simulink model "BillardSchieftischOneBall"  (Simulink 7.1)
settings: Solver=ode45  StartTime=0.0  StopTime=15.0  RelTol=1e-3
libraries: simulink x1
settings Model: Creator=Meisel  LastModifiedBy=Meisel

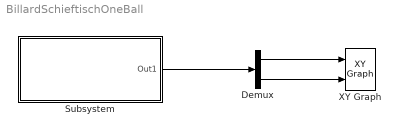
== system BillardSchieftischOneBall ==
  Demux : Demux  Outputs=2
  Subsystem : Subsystem  mask{r=0.05, x0=[0.2, 0.2], v0=[1, 1.9]}
      mask prompts: r "Ballradius"
  XY Graph : simulink/Sinks/XY Graph  SystemSampleTime=-1  xmin=0  xmax=1  ymin=0  ymax=2  st=-1
  wires:
  Subsystem/1(Out1) -> Demux/1
  Demux/1 -> XY Graph/1
  Demux/2 -> XY Graph/2

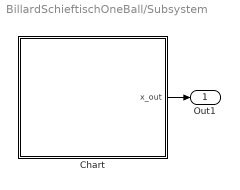
== system BillardSchieftischOneBall/Subsystem ==
  Chart : Stateflow chart
  Out1 : Outport
  wires:
  Chart/1(x_out) -> Out1/1

== stateflow chart Subsystem/Chart ==
  settings: updateMethod=CONTINUOUS
  state Roll
    during:
    // Derivatives
    x_dot=v;
    v_dot=0;
    // Output
    x_out=x;
  (default) -> Roll : {Init();}
  Roll -> Roll : [isBallOutOfBounds() != 0 ]
      | {Reflection();}
  data: fl function_output int32; r parameter double; p1 local double size=2 =0; p2 local double size=2 =0; p3 local double size=2 =0; p4 local double size=2 =0; x local double size=2; v local double size=2; x_out output double size=2; x0 parameter double size=2; v0 parameter double size=2; t local double size=4,2; n local double size=4,2; dist local double size=4
  data x settings: updateMethod=SF_CONTINUOUS_TIME_DATA
  data v settings: updateMethod=SF_CONTINUOUS_TIME_DATA
  function Init:
    | function Init
    | 
    | % Ecken des Tisches festlegen
    | p1 = [0; 0];
    | p2 = [1; 0];
    | p3 = [1; 2];
    | p4 = [0; 1];
    | 
    | x = x0; % Parameter --> Startvektor
    | v = v0; % Parameter --> Geschwindigkeitsvektor 
    | 
    | % Tangential- und Normalvektoren aller
    | % Tischseiten berechnen
    | t(1,:) = (p2-p1)/norm(p2-p1);
    | t(2,:) = (p3-p2)/norm(p3-p2);
    | t(3,:) = (p4-p3)/norm(p4-p3);
    | t(4,:) = (p1-p4)/norm(p1-p4);
    | n(1,:) = [-t(1,2), t(1,1)];
    | n(2,:) = [-t(2,2), t(2,1)];
    | n(3,:) = [-t(3,2), t(3,1)];
    | n(4,:) = [-t(4,2), t(4,1)];
  function fl = isBallOutOfBounds:
    | function fl = isBallOutOfBounds()
    | 
    | % Abstände von allen Tischseiten berechnen
    | d1 =(x-p1)'*n(1,:)';
    | d2 =(x-p2)'*n(2,:)';
    | d3 =(x-p3)'*n(3,:)';
    | d4 =(x-p4)'*n(4,:)';
    | 
    | % Kontakt mit Tischseite überprüfen
    | % fl = Tischseitennummer
    | % fl=0 : Kein Kontakt mit irgend einer Tischseite
    | if  d1 <= r
    |     fl = int32(1);
    | elseif d2 <= r
    |     fl = int32(2);
    | elseif d3 <= r
    |     fl = int32(3);
    | elseif d4 <= r
    |     fl = int32(4);
    | else
    |     fl = int32(0);
    | end
  function Reflection:
    | function Reflection
    | 
    | % Muss leider nochmal berechnet werden, da 
    | % Ergebnisübergabe aus Condition nicht möglich !
    | % Grund: Local Variables können in der Bedingungsabfrage 
    | % nicht verändert werden!
    | fl = isBallOutOfBounds();
    | 
    | % Normalkomponente umkehren
    | switch fl
    |     case 1
    |         vt = v'*t(1,:)';
    |         vn = v'*n(1,:)';
    |         v=(vt*t(1,:) - vn*n(1,:))';
    |     case 2
    |         vt = v'*t(2,:)';
    |         vn = v'*n(2,:)';
    |         v=(vt*t(2,:) - vn*n(2,:))';
    |     case 3
    |         vt = v'*t(3,:)';
    |         vn = v'*n(3,:)';
    |         v=(vt*t(3,:) - vn*n(3,:))';
    |     case 4
    |         vt = v'*t(4,:)';
    |         vn = v'*n(4,:)';
    |         v=(vt*t(4,:) - vn*n(4,:))';
    | end
